simulink model "full_maneuver_platoon_new_strategy"  (R2019a)
settings: Solver=VariableStepAuto  StartTime=0.0  StopTime=70  FixedStep=0.1  MaxStep=0.05  RelTol=1e-3
libraries: simulink x97, dspsigops x7, powerlib_meascontrol x7, autolibshared x7
(part 6 of 7)

== system full_maneuver_platoon_new_strategy/p1/Vehicle Following During LC/Velocity Control ==
  velocity : Inport
  realInput : Inport  Port=2
  intReset : Inport  Port=3
  Anti-windup gain : Gain  Gain=velKp/velKi
  Integrator2 : Integrator  ExternalReset=falling
  Sum : Sum  Inputs=|+-
  Sum1 : Sum  Inputs=|-+
  Sum2 : Sum  Inputs=-+|
  Sum3 : Sum  Inputs=|++
  freeFlowVel : Constant  Value=freeFlowVel
  velKi : Gain  Gain=velKi
  velKp : Gain  Gain=velKp
  u : Outport
  wires:
  Sum/1 -> velKi/1, velKp/1
  velKp/1 -> Sum3/2
  velKi/1 -> Sum2/2
  Integrator2/1 -> Sum3/1
  velocity/1 -> Sum/2
  freeFlowVel/1 -> Sum/1
  intReset/1 -> Integrator2/2
  Sum3/1 -> Sum1/2, u/1
  Anti-windup gain/1 -> Sum2/1
  realInput/1 -> Sum1/1
  Sum1/1 -> Anti-windup gain/1
  Sum2/1 -> Integrator2/1

== system full_maneuver_platoon_new_strategy/p1/Virtual Vehicle Following/Compute Errors ==
  xf : Inport
  vf : Inport  Port=2
  xl : Inport  Port=3
  vl : Inport  Port=4
  lcFlag : Inport  Port=5
  Compare To Constant : simulink/Logic and Bit Operations/Compare To Constant  relop=<=  const=0  OutDataTypeStr=boolean
  Demux : Demux  Outputs=2
  Demux1 : Demux  Outputs=2
  Gain3 : Gain  Gain=velFilterGain/10
  Integrator : Integrator  InitialCondition=[h d0]
  Integrator1 : Integrator  InitialCondition=vx0
  Multiply : Product
  Mux : Mux  Inputs=2
  Mux1 : Mux  Inputs=2
  Product : Product
  Saturation : Saturate  UpperLimit=maxAcceleration  LowerLimit=minAcceleration
  Sum : Sum  Inputs=-+|
  Sum1 : Sum  Inputs=++|
  Sum2 : Sum  Inputs=+-|
  Sum3 : Sum  Inputs=|++
  Sum4 : Sum  Inputs=-+|
  Sum5 : Sum  Inputs=|+-
  Sum6 : Sum  Inputs=+-|
  Sum7 : Sum  Inputs=|++
  Sum8 : Sum  Inputs=|+-
  Switch : Switch  Criteria=u2 > Threshold
  d0 : Constant  Value=d0
  d0Lc : Constant  Value=d0Lc
  h : Constant  Value=h
  hFilterGain : Gain  Gain=hFilterGain
  hLc : Constant  Value=hLc
  vLen : Constant  Value=lr+lf
  eh : Outport
  ev : Outport  Port=2
  "gap " : Outport  Port=3
  unsafeFlag : Outport  Port=4
  wires:
  vl/1 -> Sum8/1
  Saturation/1 -> Integrator1/1
  Sum8/1 -> Gain3/1
  Gain3/1 -> Saturation/1
  Integrator1/1 -> Sum8/2, Sum4/2
  Sum4/1 -> ev/1
  d0Lc/1 -> Mux1/2
  hFilterGain/1 -> Integrator/1
  Demux/1 -> Multiply/2
  xf/1 -> Sum1/2
  Sum/1 -> Sum2/1, "gap "/1, Sum6/1  "gap"
  Multiply/1 -> Sum3/1
  Demux1/2 -> Sum7/2
  hLc/1 -> Mux1/1
  vLen/1 -> Sum1/1
  Demux/2 -> Sum3/2
  Switch/1 -> Sum5/1
  Sum5/1 -> hFilterGain/1
  vf/1 -> Multiply/1, Product/1, Sum4/1
  Sum1/1 -> Sum/1  "x (front bumber)"
  Sum3/1 -> Sum2/2  "desired  gap"
  h/1 -> Mux/1
  Product/1 -> Sum7/1
  xl/1 -> Sum/2
  lcFlag/1 -> Switch/2
  Sum2/1 -> eh/1
  Compare To Constant/1 -> unsafeFlag/1
  Demux1/1 -> Product/2
  Integrator/1 -> Sum5/2, Demux/1
  d0/1 -> Mux/2
  Mux1/1 -> Switch/1
  Sum7/1 -> Sum6/2  "safe  gap"
  Mux/1 -> Switch/3, Demux1/1  "min safe gap"
  Sum6/1 -> Compare To Constant/1

== system full_maneuver_platoon_new_strategy/p1/Virtual Vehicle Following/Velocity Control ==
  note: Velocity control
  intReset : Inport
  ev : Inport  Port=2
  Integrator2 : Integrator  ExternalReset=rising
  Sum3 : Sum
  velKi : Gain  Gain=velKi
  velKp : Gain  Gain=velKp
  Out1 : Outport
  wires:
  intReset/1 -> Integrator2/2
  ev/1 -> Integrator2/1, velKp/1
  velKp/1 -> Sum3/1
  Sum3/1 -> Out1/1
  velKi/1 -> Sum3/2
  Integrator2/1 -> velKi/1

== system full_maneuver_platoon_new_strategy/p1/Virtual Vehicle Following/Virtual Leader Following ==
  eh : Inport
  ev : Inport  Port=2
  realInput : Inport  Port=3
  Anti-windup gain : Gain  Gain=sqrt(Ki/Kd)
  Integrator : Integrator
  Kd : Gain  Gain=Kd
  Ki : Gain  Gain=Ki
  Kp : Gain  Gain=Kp
  Saturation1 : Saturate  UpperLimit=maxHeadwayError  LowerLimit=minHeadwayError
  Scope : Scope  NumInputPorts=4
  Sum : Sum  Inputs=|-+
  Sum1 : Sum  Inputs=+++
  Sum5 : Sum  Inputs=-+|
  u : Outport
  wires:
  Sum/1 -> Anti-windup gain/1
  realInput/1 -> Sum/1
  Sum1/1 -> u/1, Sum/2, Scope/4
  eh/1 -> Saturation1/1
  Saturation1/1 -> Ki/1, Kp/1
  Kd/1 -> Sum1/3, Scope/3
  Kp/1 -> Sum1/2, Scope/2
  Integrator/1 -> Sum1/1, Scope/1
  Sum5/1 -> Integrator/1
  Anti-windup gain/1 -> Sum5/1
  Ki/1 -> Sum5/2
  ev/1 -> Kd/1

== system full_maneuver_platoon_new_strategy/p1/followerErrors/gapToFollower ==
  xf : Inport
  vf : Inport  Port=2
  xl : Inport  Port=3
  Multiply : Product
  Sum : Sum  Inputs=-+|
  Sum1 : Sum  Inputs=++|
  Sum2 : Sum  Inputs=+-|
  Sum3 : Sum  Inputs=|++
  d0 : Constant  Value=d0
  h : Constant  Value=h
  vLen : Constant  Value=lr+lf
  eh : Outport
  "gap " : Outport  Port=2
  wires:
  d0/1 -> Sum3/2  "gap at  standstill"
  h/1 -> Multiply/2  "time headway"
  Sum2/1 -> eh/1
  xl/1 -> Sum/2
  Sum1/1 -> Sum/1  "x (front bumber)"
  vf/1 -> Multiply/1
  Sum3/1 -> Sum2/2  "desired  gap"
  xf/1 -> Sum1/2
  Sum/1 -> Sum2/1, "gap "/1  "gap"
  Multiply/1 -> Sum3/1
  vLen/1 -> Sum1/1

== system full_maneuver_platoon_new_strategy/p2/Lateral Control/Full State Observer ==
  note: yhat
  note: xhat
  measuredOutputs : Inport
  delta : Inport  Port=2
  Add1 : Sum  Inputs=|-+
  Gain : Gain  Gain=B  Multiplication=Matrix(K*u)
  Gain1 : Gain  Gain=C  Multiplication=Matrix(K*u)
  Gain2 : Gain  Gain=L  Multiplication=Matrix(K*u)
  Gain3 : Gain  Gain=A  Multiplication=Matrix(K*u)
  Integrator : Integrator  InitialCondition=[y0; 0; 0; 0]
  Signal Specification : SignalSpecification  Dimensions=[size(C,1) 1]
  Sum : Sum  Inputs=+++
  xhat : Outport
  wires:
  Gain2/1 -> Sum/1
  Signal Specification/1 -> Gain2/1
  Gain3/1 -> Sum/2
  Gain/1 -> Sum/3
  delta/1 -> Gain/1
  measuredOutputs/1 -> Add1/2
  Sum/1 -> Integrator/1
  Gain1/1 -> Add1/1
  Integrator/1 -> Gain1/1, Gain3/1, xhat/1
  Add1/1 -> Signal Specification/1

== system full_maneuver_platoon_new_strategy/p2/Lateral Control/Triggered Subsystem1 ==
  In1 : Inport
  Trigger : TriggerPort  VariantControl=Variant
  Out1 : Outport  InitialOutput=y0
  wires:
  In1/1 -> Out1/1

== system full_maneuver_platoon_new_strategy/p2/Regular Vehicle Following/Compute Errors ==
  xf : Inport
  vf : Inport  Port=2
  xl : Inport  Port=3
  vl : Inport  Port=4
  extraSpaceFlag : Inport  Port=5
  Compare To Constant : simulink/Logic and Bit Operations/Compare To Constant  relop=<  const=-0.1  OutDataTypeStr=boolean
  Demux : Demux  Outputs=2
  Demux1 : Demux  Outputs=2
  Gain3 : Gain  Gain=velFilterGain
  Integrator : Integrator  InitialCondition=[h d0]
  Integrator1 : Integrator  InitialCondition=vx0
  Multiply : Product
  Mux : Mux  Inputs=2
  Mux1 : Mux  Inputs=2
  Product : Product
  Saturation : Saturate  UpperLimit=maxAcceleration  LowerLimit=minAcceleration
  Sum : Sum  Inputs=-+|
  Sum1 : Sum  Inputs=++|
  Sum2 : Sum  Inputs=+-|
  Sum3 : Sum  Inputs=|++
  Sum4 : Sum  Inputs=-+|
  Sum5 : Sum  Inputs=|+-
  Sum6 : Sum  Inputs=+-|
  Sum7 : Sum  Inputs=|++
  Sum8 : Sum  Inputs=|+-
  Switch : Switch  Criteria=u2 > Threshold
  d0 : Constant  Value=d0
  d0Lc : Constant  Value=d0Lc
  h : Constant  Value=h
  hFilterGain : Gain  Gain=hFilterGain
  hLc : Constant  Value=hLc
  vLen : Constant  Value=lr+lf
  eh : Outport
  ev : Outport  Port=2
  "gap " : Outport  Port=3
  unsafeFlag : Outport  Port=4
  wires:
  Sum6/1 -> Compare To Constant/1
  Mux/1 -> Switch/3, Demux1/1  "min safe gap"
  Sum7/1 -> Sum6/2  "safe  gap"
  Mux1/1 -> Switch/1
  d0/1 -> Mux/2
  Integrator/1 -> Demux/1, Sum5/2
  Demux1/1 -> Product/2
  Compare To Constant/1 -> unsafeFlag/1
  Sum2/1 -> eh/1
  extraSpaceFlag/1 -> Switch/2
  xl/1 -> Sum/2
  Product/1 -> Sum7/1
  h/1 -> Mux/1
  Sum3/1 -> Sum2/2  "desired  gap"
  Sum1/1 -> Sum/1  "x (front bumber)"
  vf/1 -> Sum4/1, Product/1, Multiply/1
  Sum5/1 -> hFilterGain/1
  Switch/1 -> Sum5/1
  Demux/2 -> Sum3/2
  vLen/1 -> Sum1/1
  hLc/1 -> Mux1/1
  Demux1/2 -> Sum7/2
  Multiply/1 -> Sum3/1
  Sum/1 -> Sum6/1, "gap "/1, Sum2/1  "gap"
  xf/1 -> Sum1/2
  Demux/1 -> Multiply/2
  hFilterGain/1 -> Integrator/1
  d0Lc/1 -> Mux1/2
  vl/1 -> Sum8/1
  Sum4/1 -> ev/1
  Gain3/1 -> Saturation/1
  Saturation/1 -> Integrator1/1
  Integrator1/1 -> Sum4/2, Sum8/2
  Sum8/1 -> Gain3/1

== system full_maneuver_platoon_new_strategy/p2/Regular Vehicle Following/Free Flow Velocity Control ==
  ev : Inport
  realInput : Inport  Port=2
  intReset : Inport  Port=3
  Anti-windup gain : Gain  Gain=velKp/velKi
  Integrator2 : Integrator  ExternalReset=falling
  Sum1 : Sum  Inputs=|-+
  Sum2 : Sum  Inputs=-+|
  Sum3 : Sum  Inputs=|++
  velKi : Gain  Gain=velKi
  velKp : Gain  Gain=velKp
  u : Outport
  wires:
  ev/1 -> velKp/1, velKi/1
  velKp/1 -> Sum3/2
  velKi/1 -> Sum2/2
  Integrator2/1 -> Sum3/1
  intReset/1 -> Integrator2/2
  Sum3/1 -> Sum1/2, u/1
  Anti-windup gain/1 -> Sum2/1
  realInput/1 -> Sum1/1
  Sum1/1 -> Anti-windup gain/1
  Sum2/1 -> Integrator2/1

== system full_maneuver_platoon_new_strategy/p2/Regular Vehicle Following/Minimum Velocity Control ==
  ev : Inport
  realInput : Inport  Port=2
  intReset : Inport  Port=3
  Anti-windup gain : Gain  Gain=velKp/velKi
  Integrator2 : Integrator  ExternalReset=rising
  Sum1 : Sum  Inputs=|-+
  Sum2 : Sum  Inputs=-+|
  Sum3 : Sum  Inputs=|++
  velKi : Gain  Gain=velKi
  velKp : Gain  Gain=velKp
  u : Outport
  wires:
  ev/1 -> velKp/1, velKi/1
  velKp/1 -> Sum3/2
  velKi/1 -> Sum2/2
  Integrator2/1 -> Sum3/1
  intReset/1 -> Integrator2/2
  Sum3/1 -> Sum1/2, u/1
  Anti-windup gain/1 -> Sum2/1
  realInput/1 -> Sum1/1
  Sum1/1 -> Anti-windup gain/1
  Sum2/1 -> Integrator2/1

== system full_maneuver_platoon_new_strategy/p2/Regular Vehicle Following/Veh Following ==
  eh : Inport
  ev : Inport  Port=2
  realInput : Inport  Port=3
  intReset : Inport  Port=4
  Anti-windup gain : Gain  Gain=sqrt(Ki/Kd)
  Integrator : Integrator  ExternalReset=rising
  Kd : Gain  Gain=Kd
  Ki : Gain  Gain=Ki
  Kp : Gain  Gain=Kp
  Saturation1 : Saturate  UpperLimit=maxHeadwayError  LowerLimit=minHeadwayError
  Scope : Scope  NumInputPorts=4
  Sum : Sum  Inputs=|-+
  Sum1 : Sum  Inputs=+++
  Sum5 : Sum  Inputs=-+|
  u : Outport
  wires:
  ev/1 -> Kd/1
  Ki/1 -> Sum5/2
  Anti-windup gain/1 -> Sum5/1
  Sum5/1 -> Integrator/1
  Integrator/1 -> Sum1/1, Scope/1
  Kp/1 -> Sum1/2, Scope/2
  Kd/1 -> Scope/3, Sum1/3
  Saturation1/1 -> Kp/1, Ki/1
  eh/1 -> Saturation1/1
  Sum1/1 -> Sum/2, u/1, Scope/4
  realInput/1 -> Sum/1
  Sum/1 -> Anti-windup gain/1
  intReset/1 -> Integrator/2

== system full_maneuver_platoon_new_strategy/p2/Vehicle Following During LC/Compute Errors ==
  xf : Inport
  vf : Inport  Port=2
  xl : Inport  Port=3
  vl : Inport  Port=4
  extraSpaceFlag : Inport  Port=5
  Compare To Constant : simulink/Logic and Bit Operations/Compare To Constant  relop=<=  const=0  OutDataTypeStr=boolean
  Demux : Demux  Outputs=2
  Demux1 : Demux  Outputs=2
  Gain3 : Gain  Gain=velFilterGain
  Integrator : Integrator  InitialCondition=[h d0]
  Integrator1 : Integrator  InitialCondition=vx0
  Multiply : Product
  Mux : Mux  Inputs=2
  Mux1 : Mux  Inputs=2
  Product : Product
  Saturation : Saturate  UpperLimit=maxAcceleration  LowerLimit=minAcceleration
  Sum : Sum  Inputs=-+|
  Sum1 : Sum  Inputs=++|
  Sum2 : Sum  Inputs=+-|
  Sum3 : Sum  Inputs=|++
  Sum4 : Sum  Inputs=-+|
  Sum5 : Sum  Inputs=|+-
  Sum6 : Sum  Inputs=+-|
  Sum7 : Sum  Inputs=|++
  Sum8 : Sum  Inputs=|+-
  Switch : Switch  Criteria=u2 > Threshold
  d0 : Constant  Value=d0
  d0Lc : Constant  Value=d0Lc
  h : Constant  Value=h
  hFilterGain : Gain  Gain=hFilterGain
  hLc : Constant  Value=hLc
  vLen : Constant  Value=lr+lf
  eh : Outport
  ev : Outport  Port=2
  "gap " : Outport  Port=3
  unsafeFlag : Outport  Port=4
  wires:
  Sum4/1 -> ev/1
  d0Lc/1 -> Mux1/2
  hFilterGain/1 -> Integrator/1
  Demux/1 -> Multiply/2
  xf/1 -> Sum1/2
  Sum/1 -> Sum2/1, "gap "/1, Sum6/1  "gap"
  Multiply/1 -> Sum3/1
  Demux1/2 -> Sum7/2
  hLc/1 -> Mux1/1
  vLen/1 -> Sum1/1
  Demux/2 -> Sum3/2
  Switch/1 -> Sum5/1
  Sum5/1 -> hFilterGain/1
  vf/1 -> Multiply/1, Product/1, Sum4/1
  Sum1/1 -> Sum/1  "x (front bumber)"
  Sum3/1 -> Sum2/2  "desired  gap"
  h/1 -> Mux/1
  Product/1 -> Sum7/1
  xl/1 -> Sum/2
  extraSpaceFlag/1 -> Switch/2
  Sum2/1 -> eh/1
  Compare To Constant/1 -> unsafeFlag/1
  Demux1/1 -> Product/2
  Integrator/1 -> Sum5/2, Demux/1
  d0/1 -> Mux/2
  Mux1/1 -> Switch/1
  Sum7/1 -> Sum6/2  "safe  gap"
  Mux/1 -> Switch/3, Demux1/1  "min safe gap"
  Sum6/1 -> Compare To Constant/1
  Saturation/1 -> Integrator1/1
  Gain3/1 -> Saturation/1
  Integrator1/1 -> Sum4/2, Sum8/2
  Sum8/1 -> Gain3/1
  vl/1 -> Sum8/1

== system full_maneuver_platoon_new_strategy/p2/Vehicle Following During LC/Veh Following ==
  eh : Inport
  ev : Inport  Port=2
  realInput : Inport  Port=3
  intReset : Inport  Port=4
  Anti-windup gain : Gain  Gain=sqrt(Ki/Kd)
  Integrator : Integrator  ExternalReset=rising
  Kd : Gain  Gain=Kd
  Ki : Gain  Gain=Ki
  Kp : Gain  Gain=Kp
  Saturation1 : Saturate  UpperLimit=maxHeadwayError  LowerLimit=minHeadwayError
  Scope : Scope  NumInputPorts=4
  Sum : Sum  Inputs=|-+
  Sum1 : Sum  Inputs=+++
  Sum5 : Sum  Inputs=-+|
  u : Outport
  wires:
  intReset/1 -> Integrator/2
  Sum/1 -> Anti-windup gain/1
  realInput/1 -> Sum/1
  Sum1/1 -> Scope/4, u/1, Sum/2
  eh/1 -> Saturation1/1
  Saturation1/1 -> Ki/1, Kp/1
  Kd/1 -> Sum1/3, Scope/3
  Kp/1 -> Scope/2, Sum1/2
  Integrator/1 -> Scope/1, Sum1/1
  Sum5/1 -> Integrator/1
  Anti-windup gain/1 -> Sum5/1
  Ki/1 -> Sum5/2
  ev/1 -> Kd/1

== system full_maneuver_platoon_new_strategy/p2/Vehicle Following During LC/Velocity Control ==
  velocity : Inport
  realInput : Inport  Port=2
  intReset : Inport  Port=3
  Anti-windup gain : Gain  Gain=velKp/velKi
  Integrator2 : Integrator  ExternalReset=falling
  Sum : Sum  Inputs=|+-
  Sum1 : Sum  Inputs=|-+
  Sum2 : Sum  Inputs=-+|
  Sum3 : Sum  Inputs=|++
  freeFlowVel : Constant  Value=freeFlowVel
  velKi : Gain  Gain=velKi
  velKp : Gain  Gain=velKp
  u : Outport
  wires:
  Sum2/1 -> Integrator2/1
  Sum1/1 -> Anti-windup gain/1
  realInput/1 -> Sum1/1
  Anti-windup gain/1 -> Sum2/1
  Sum3/1 -> u/1, Sum1/2
  intReset/1 -> Integrator2/2
  freeFlowVel/1 -> Sum/1
  velocity/1 -> Sum/2
  Integrator2/1 -> Sum3/1
  velKi/1 -> Sum2/2
  velKp/1 -> Sum3/2
  Sum/1 -> velKp/1, velKi/1

== system full_maneuver_platoon_new_strategy/p2/Virtual Vehicle Following/Compute Errors ==
  xf : Inport
  vf : Inport  Port=2
  xl : Inport  Port=3
  vl : Inport  Port=4
  lcFlag : Inport  Port=5
  Compare To Constant : simulink/Logic and Bit Operations/Compare To Constant  relop=<=  const=0  OutDataTypeStr=boolean
  Demux : Demux  Outputs=2
  Demux1 : Demux  Outputs=2
  Gain3 : Gain  Gain=velFilterGain/10
  Integrator : Integrator  InitialCondition=[h d0]
  Integrator1 : Integrator  InitialCondition=vx0
  Multiply : Product
  Mux : Mux  Inputs=2
  Mux1 : Mux  Inputs=2
  Product : Product
  Saturation : Saturate  UpperLimit=maxAcceleration  LowerLimit=minAcceleration
  Sum : Sum  Inputs=-+|
  Sum1 : Sum  Inputs=++|
  Sum2 : Sum  Inputs=+-|
  Sum3 : Sum  Inputs=|++
  Sum4 : Sum  Inputs=-+|
  Sum5 : Sum  Inputs=|+-
  Sum6 : Sum  Inputs=+-|
  Sum7 : Sum  Inputs=|++
  Sum8 : Sum  Inputs=|+-
  Switch : Switch  Criteria=u2 > Threshold
  d0 : Constant  Value=d0
  d0Lc : Constant  Value=d0Lc
  h : Constant  Value=h
  hFilterGain : Gain  Gain=hFilterGain
  hLc : Constant  Value=hLc
  vLen : Constant  Value=lr+lf
  eh : Outport
  ev : Outport  Port=2
  "gap " : Outport  Port=3
  unsafeFlag : Outport  Port=4
  wires:
  Sum6/1 -> Compare To Constant/1
  Mux/1 -> Demux1/1, Switch/3  "min safe gap"
  Sum7/1 -> Sum6/2  "safe  gap"
  Mux1/1 -> Switch/1
  d0/1 -> Mux/2
  Integrator/1 -> Demux/1, Sum5/2
  Demux1/1 -> Product/2
  Compare To Constant/1 -> unsafeFlag/1
  Sum2/1 -> eh/1
  lcFlag/1 -> Switch/2
  xl/1 -> Sum/2
  Product/1 -> Sum7/1
  h/1 -> Mux/1
  Sum3/1 -> Sum2/2  "desired  gap"
  Sum1/1 -> Sum/1  "x (front bumber)"
  vf/1 -> Sum4/1, Product/1, Multiply/1
  Sum5/1 -> hFilterGain/1
  Switch/1 -> Sum5/1
  Demux/2 -> Sum3/2
  vLen/1 -> Sum1/1
  hLc/1 -> Mux1/1
  Demux1/2 -> Sum7/2
  Multiply/1 -> Sum3/1
  Sum/1 -> Sum6/1, "gap "/1, Sum2/1  "gap"
  xf/1 -> Sum1/2
  Demux/1 -> Multiply/2
  hFilterGain/1 -> Integrator/1
  d0Lc/1 -> Mux1/2
  Sum4/1 -> ev/1
  Integrator1/1 -> Sum4/2, Sum8/2
  Gain3/1 -> Saturation/1
  Sum8/1 -> Gain3/1
  Saturation/1 -> Integrator1/1
  vl/1 -> Sum8/1

== system full_maneuver_platoon_new_strategy/p2/Virtual Vehicle Following/Velocity Control ==
  note: Velocity control
  intReset : Inport
  ev : Inport  Port=2
  Integrator2 : Integrator  ExternalReset=rising
  Sum3 : Sum
  velKi : Gain  Gain=velKi
  velKp : Gain  Gain=velKp
  Out1 : Outport
  wires:
  Integrator2/1 -> velKi/1
  velKi/1 -> Sum3/2
  Sum3/1 -> Out1/1
  velKp/1 -> Sum3/1
  ev/1 -> velKp/1, Integrator2/1
  intReset/1 -> Integrator2/2

== system full_maneuver_platoon_new_strategy/p2/Virtual Vehicle Following/Virtual Leader Following ==
  eh : Inport
  ev : Inport  Port=2
  realInput : Inport  Port=3
  Anti-windup gain : Gain  Gain=sqrt(Ki/Kd)
  Integrator : Integrator
  Kd : Gain  Gain=Kd
  Ki : Gain  Gain=Ki
  Kp : Gain  Gain=Kp
  Saturation1 : Saturate  UpperLimit=maxHeadwayError  LowerLimit=minHeadwayError
  Scope : Scope  NumInputPorts=4
  Sum : Sum  Inputs=|-+
  Sum1 : Sum  Inputs=+++
  Sum5 : Sum  Inputs=-+|
  u : Outport
  wires:
  ev/1 -> Kd/1
  Ki/1 -> Sum5/2
  Anti-windup gain/1 -> Sum5/1
  Sum5/1 -> Integrator/1
  Integrator/1 -> Scope/1, Sum1/1
  Kp/1 -> Scope/2, Sum1/2
  Kd/1 -> Scope/3, Sum1/3
  Saturation1/1 -> Kp/1, Ki/1
  eh/1 -> Saturation1/1
  Sum1/1 -> Scope/4, Sum/2, u/1
  realInput/1 -> Sum/1
  Sum/1 -> Anti-windup gain/1

== system full_maneuver_platoon_new_strategy/p2/followerErrors/gapToFollower ==
  xf : Inport
  vf : Inport  Port=2
  xl : Inport  Port=3
  Multiply : Product
  Sum : Sum  Inputs=-+|
  Sum1 : Sum  Inputs=++|
  Sum2 : Sum  Inputs=+-|
  Sum3 : Sum  Inputs=|++
  d0 : Constant  Value=d0
  h : Constant  Value=h
  vLen : Constant  Value=lr+lf
  eh : Outport
  "gap " : Outport  Port=2
  wires:
  vLen/1 -> Sum1/1
  Multiply/1 -> Sum3/1
  Sum/1 -> "gap "/1, Sum2/1  "gap"
  xf/1 -> Sum1/2
  Sum3/1 -> Sum2/2  "desired  gap"
  vf/1 -> Multiply/1
  Sum1/1 -> Sum/1  "x (front bumber)"
  xl/1 -> Sum/2
  Sum2/1 -> eh/1
  h/1 -> Multiply/2  "time headway"
  d0/1 -> Sum3/2  "gap at  standstill"

== system full_maneuver_platoon_new_strategy/p3/Lateral Control/Full State Observer ==
  note: xhat
  note: yhat
  measuredOutputs : Inport
  delta : Inport  Port=2
  Add1 : Sum  Inputs=|-+
  Gain : Gain  Gain=B  Multiplication=Matrix(K*u)
  Gain1 : Gain  Gain=C  Multiplication=Matrix(K*u)
  Gain2 : Gain  Gain=L  Multiplication=Matrix(K*u)
  Gain3 : Gain  Gain=A  Multiplication=Matrix(K*u)
  Integrator : Integrator  InitialCondition=[y0; 0; 0; 0]
  Signal Specification : SignalSpecification  Dimensions=[size(C,1) 1]
  Sum : Sum  Inputs=+++
  xhat : Outport
  wires:
  Add1/1 -> Signal Specification/1
  Integrator/1 -> xhat/1, Gain3/1, Gain1/1
  Gain1/1 -> Add1/1
  Sum/1 -> Integrator/1
  measuredOutputs/1 -> Add1/2
  delta/1 -> Gain/1
  Gain/1 -> Sum/3
  Gain3/1 -> Sum/2
  Signal Specification/1 -> Gain2/1
  Gain2/1 -> Sum/1

== system full_maneuver_platoon_new_strategy/p3/Lateral Control/Triggered Subsystem1 ==
  In1 : Inport
  Trigger : TriggerPort  VariantControl=Variant
  Out1 : Outport  InitialOutput=y0
  wires:
  In1/1 -> Out1/1

== system full_maneuver_platoon_new_strategy/p3/Regular Vehicle Following/Compute Errors ==
  xf : Inport
  vf : Inport  Port=2
  xl : Inport  Port=3
  vl : Inport  Port=4
  extraSpaceFlag : Inport  Port=5
  Compare To Constant : simulink/Logic and Bit Operations/Compare To Constant  relop=<  const=-0.1  OutDataTypeStr=boolean
  Demux : Demux  Outputs=2
  Demux1 : Demux  Outputs=2
  Gain3 : Gain  Gain=velFilterGain
  Integrator : Integrator  InitialCondition=[h d0]
  Integrator1 : Integrator  InitialCondition=vx0
  Multiply : Product
  Mux : Mux  Inputs=2
  Mux1 : Mux  Inputs=2
  Product : Product
  Saturation : Saturate  UpperLimit=maxAcceleration  LowerLimit=minAcceleration
  Sum : Sum  Inputs=-+|
  Sum1 : Sum  Inputs=++|
  Sum2 : Sum  Inputs=+-|
  Sum3 : Sum  Inputs=|++
  Sum4 : Sum  Inputs=-+|
  Sum5 : Sum  Inputs=|+-
  Sum6 : Sum  Inputs=+-|
  Sum7 : Sum  Inputs=|++
  Sum8 : Sum  Inputs=|+-
  Switch : Switch  Criteria=u2 > Threshold
  d0 : Constant  Value=d0
  d0Lc : Constant  Value=d0Lc
  h : Constant  Value=h
  hFilterGain : Gain  Gain=hFilterGain
  hLc : Constant  Value=hLc
  vLen : Constant  Value=lr+lf
  eh : Outport
  ev : Outport  Port=2
  "gap " : Outport  Port=3
  unsafeFlag : Outport  Port=4
  wires:
  Sum8/1 -> Gain3/1
  Integrator1/1 -> Sum8/2, Sum4/2
  Saturation/1 -> Integrator1/1
  Gain3/1 -> Saturation/1
  Sum4/1 -> ev/1
  vl/1 -> Sum8/1
  d0Lc/1 -> Mux1/2
  hFilterGain/1 -> Integrator/1
  Demux/1 -> Multiply/2
  xf/1 -> Sum1/2
  Sum/1 -> Sum2/1, "gap "/1, Sum6/1  "gap"
  Multiply/1 -> Sum3/1
  Demux1/2 -> Sum7/2
  hLc/1 -> Mux1/1
  vLen/1 -> Sum1/1
  Demux/2 -> Sum3/2
  Switch/1 -> Sum5/1
  Sum5/1 -> hFilterGain/1
  vf/1 -> Multiply/1, Product/1, Sum4/1
  Sum1/1 -> Sum/1  "x (front bumber)"
  Sum3/1 -> Sum2/2  "desired  gap"
  h/1 -> Mux/1
  Product/1 -> Sum7/1
  xl/1 -> Sum/2
  extraSpaceFlag/1 -> Switch/2
  Sum2/1 -> eh/1
  Compare To Constant/1 -> unsafeFlag/1
  Demux1/1 -> Product/2
  Integrator/1 -> Sum5/2, Demux/1
  d0/1 -> Mux/2
  Mux1/1 -> Switch/1
  Sum7/1 -> Sum6/2  "safe  gap"
  Mux/1 -> Demux1/1, Switch/3  "min safe gap"
  Sum6/1 -> Compare To Constant/1

== system full_maneuver_platoon_new_strategy/p3/Regular Vehicle Following/Free Flow Velocity Control ==
  ev : Inport
  realInput : Inport  Port=2
  intReset : Inport  Port=3
  Anti-windup gain : Gain  Gain=velKp/velKi
  Integrator2 : Integrator  ExternalReset=falling
  Sum1 : Sum  Inputs=|-+
  Sum2 : Sum  Inputs=-+|
  Sum3 : Sum  Inputs=|++
  velKi : Gain  Gain=velKi
  velKp : Gain  Gain=velKp
  u : Outport
  wires:
  Sum2/1 -> Integrator2/1
  Sum1/1 -> Anti-windup gain/1
  realInput/1 -> Sum1/1
  Anti-windup gain/1 -> Sum2/1
  Sum3/1 -> u/1, Sum1/2
  intReset/1 -> Integrator2/2
  Integrator2/1 -> Sum3/1
  velKi/1 -> Sum2/2
  velKp/1 -> Sum3/2
  ev/1 -> velKi/1, velKp/1

== system full_maneuver_platoon_new_strategy/p3/Regular Vehicle Following/Minimum Velocity Control ==
  ev : Inport
  realInput : Inport  Port=2
  intReset : Inport  Port=3
  Anti-windup gain : Gain  Gain=velKp/velKi
  Integrator2 : Integrator  ExternalReset=rising
  Sum1 : Sum  Inputs=|-+
  Sum2 : Sum  Inputs=-+|
  Sum3 : Sum  Inputs=|++
  velKi : Gain  Gain=velKi
  velKp : Gain  Gain=velKp
  u : Outport
  wires:
  Sum2/1 -> Integrator2/1
  Sum1/1 -> Anti-windup gain/1
  realInput/1 -> Sum1/1
  Anti-windup gain/1 -> Sum2/1
  Sum3/1 -> u/1, Sum1/2
  intReset/1 -> Integrator2/2
  Integrator2/1 -> Sum3/1
  velKi/1 -> Sum2/2
  velKp/1 -> Sum3/2
  ev/1 -> velKi/1, velKp/1

== system full_maneuver_platoon_new_strategy/p3/Regular Vehicle Following/Veh Following ==
  eh : Inport
  ev : Inport  Port=2
  realInput : Inport  Port=3
  intReset : Inport  Port=4
  Anti-windup gain : Gain  Gain=sqrt(Ki/Kd)
  Integrator : Integrator  ExternalReset=rising
  Kd : Gain  Gain=Kd
  Ki : Gain  Gain=Ki
  Kp : Gain  Gain=Kp
  Saturation1 : Saturate  UpperLimit=maxHeadwayError  LowerLimit=minHeadwayError
  Scope : Scope  NumInputPorts=4
  Sum : Sum  Inputs=|-+
  Sum1 : Sum  Inputs=+++
  Sum5 : Sum  Inputs=-+|
  u : Outport
  wires:
  intReset/1 -> Integrator/2
  Sum/1 -> Anti-windup gain/1
  realInput/1 -> Sum/1
  Sum1/1 -> Scope/4, u/1, Sum/2
  eh/1 -> Saturation1/1
  Saturation1/1 -> Ki/1, Kp/1
  Kd/1 -> Sum1/3, Scope/3
  Kp/1 -> Scope/2, Sum1/2
  Integrator/1 -> Scope/1, Sum1/1
  Sum5/1 -> Integrator/1
  Anti-windup gain/1 -> Sum5/1
  Ki/1 -> Sum5/2
  ev/1 -> Kd/1

== system full_maneuver_platoon_new_strategy/p3/Vehicle Following During LC/Compute Errors ==
  xf : Inport
  vf : Inport  Port=2
  xl : Inport  Port=3
  vl : Inport  Port=4
  extraSpaceFlag : Inport  Port=5
  Compare To Constant : simulink/Logic and Bit Operations/Compare To Constant  relop=<=  const=0  OutDataTypeStr=boolean
  Demux : Demux  Outputs=2
  Demux1 : Demux  Outputs=2
  Gain3 : Gain  Gain=velFilterGain
  Integrator : Integrator  InitialCondition=[h d0]
  Integrator1 : Integrator  InitialCondition=vx0
  Multiply : Product
  Mux : Mux  Inputs=2
  Mux1 : Mux  Inputs=2
  Product : Product
  Saturation : Saturate  UpperLimit=maxAcceleration  LowerLimit=minAcceleration
  Sum : Sum  Inputs=-+|
  Sum1 : Sum  Inputs=++|
  Sum2 : Sum  Inputs=+-|
  Sum3 : Sum  Inputs=|++
  Sum4 : Sum  Inputs=-+|
  Sum5 : Sum  Inputs=|+-
  Sum6 : Sum  Inputs=+-|
  Sum7 : Sum  Inputs=|++
  Sum8 : Sum  Inputs=|+-
  Switch : Switch  Criteria=u2 > Threshold
  d0 : Constant  Value=d0
  d0Lc : Constant  Value=d0Lc
  h : Constant  Value=h
  hFilterGain : Gain  Gain=hFilterGain
  hLc : Constant  Value=hLc
  vLen : Constant  Value=lr+lf
  eh : Outport
  ev : Outport  Port=2
  "gap " : Outport  Port=3
  unsafeFlag : Outport  Port=4
  wires:
  vl/1 -> Sum8/1
  Sum8/1 -> Gain3/1
  Integrator1/1 -> Sum8/2, Sum4/2
  Gain3/1 -> Saturation/1
  Saturation/1 -> Integrator1/1
  Sum6/1 -> Compare To Constant/1
  Mux/1 -> Demux1/1, Switch/3  "min safe gap"
  Sum7/1 -> Sum6/2  "safe  gap"
  Mux1/1 -> Switch/1
  d0/1 -> Mux/2
  Integrator/1 -> Demux/1, Sum5/2
  Demux1/1 -> Product/2
  Compare To Constant/1 -> unsafeFlag/1
  Sum2/1 -> eh/1
  extraSpaceFlag/1 -> Switch/2
  xl/1 -> Sum/2
  Product/1 -> Sum7/1
  h/1 -> Mux/1
  Sum3/1 -> Sum2/2  "desired  gap"
  Sum1/1 -> Sum/1  "x (front bumber)"
  vf/1 -> Sum4/1, Product/1, Multiply/1
  Sum5/1 -> hFilterGain/1
  Switch/1 -> Sum5/1
  Demux/2 -> Sum3/2
  vLen/1 -> Sum1/1
  hLc/1 -> Mux1/1
  Demux1/2 -> Sum7/2
  Multiply/1 -> Sum3/1
  Sum/1 -> Sum6/1, "gap "/1, Sum2/1  "gap"
  xf/1 -> Sum1/2
  Demux/1 -> Multiply/2
  hFilterGain/1 -> Integrator/1
  d0Lc/1 -> Mux1/2
  Sum4/1 -> ev/1

== system full_maneuver_platoon_new_strategy/p3/Vehicle Following During LC/Veh Following ==
  eh : Inport
  ev : Inport  Port=2
  realInput : Inport  Port=3
  intReset : Inport  Port=4
  Anti-windup gain : Gain  Gain=sqrt(Ki/Kd)
  Integrator : Integrator  ExternalReset=rising
  Kd : Gain  Gain=Kd
  Ki : Gain  Gain=Ki
  Kp : Gain  Gain=Kp
  Saturation1 : Saturate  UpperLimit=maxHeadwayError  LowerLimit=minHeadwayError
  Scope : Scope  NumInputPorts=4
  Sum : Sum  Inputs=|-+
  Sum1 : Sum  Inputs=+++
  Sum5 : Sum  Inputs=-+|
  u : Outport
  wires:
  ev/1 -> Kd/1
  Ki/1 -> Sum5/2
  Anti-windup gain/1 -> Sum5/1
  Sum5/1 -> Integrator/1
  Integrator/1 -> Sum1/1, Scope/1
  Kp/1 -> Sum1/2, Scope/2
  Kd/1 -> Scope/3, Sum1/3
  Saturation1/1 -> Kp/1, Ki/1
  eh/1 -> Saturation1/1
  Sum1/1 -> Sum/2, u/1, Scope/4
  realInput/1 -> Sum/1
  Sum/1 -> Anti-windup gain/1
  intReset/1 -> Integrator/2

== system full_maneuver_platoon_new_strategy/p3/Vehicle Following During LC/Velocity Control ==
  velocity : Inport
  realInput : Inport  Port=2
  intReset : Inport  Port=3
  Anti-windup gain : Gain  Gain=velKp/velKi
  Integrator2 : Integrator  ExternalReset=falling
  Sum : Sum  Inputs=|+-
  Sum1 : Sum  Inputs=|-+
  Sum2 : Sum  Inputs=-+|
  Sum3 : Sum  Inputs=|++
  freeFlowVel : Constant  Value=freeFlowVel
  velKi : Gain  Gain=velKi
  velKp : Gain  Gain=velKp
  u : Outport
  wires:
  Sum/1 -> velKi/1, velKp/1
  velKp/1 -> Sum3/2
  velKi/1 -> Sum2/2
  Integrator2/1 -> Sum3/1
  velocity/1 -> Sum/2
  freeFlowVel/1 -> Sum/1
  intReset/1 -> Integrator2/2
  Sum3/1 -> Sum1/2, u/1
  Anti-windup gain/1 -> Sum2/1
  realInput/1 -> Sum1/1
  Sum1/1 -> Anti-windup gain/1
  Sum2/1 -> Integrator2/1

== system full_maneuver_platoon_new_strategy/p3/Virtual Vehicle Following/Compute Errors ==
  xf : Inport
  vf : Inport  Port=2
  xl : Inport  Port=3
  vl : Inport  Port=4
  lcFlag : Inport  Port=5
  Compare To Constant : simulink/Logic and Bit Operations/Compare To Constant  relop=<=  const=0  OutDataTypeStr=boolean
  Demux : Demux  Outputs=2
  Demux1 : Demux  Outputs=2
  Gain3 : Gain  Gain=velFilterGain/10
  Integrator : Integrator  InitialCondition=[h d0]
  Integrator1 : Integrator  InitialCondition=vx0
  Multiply : Product
  Mux : Mux  Inputs=2
  Mux1 : Mux  Inputs=2
  Product : Product
  Saturation : Saturate  UpperLimit=maxAcceleration  LowerLimit=minAcceleration
  Sum : Sum  Inputs=-+|
  Sum1 : Sum  Inputs=++|
  Sum2 : Sum  Inputs=+-|
  Sum3 : Sum  Inputs=|++
  Sum4 : Sum  Inputs=-+|
  Sum5 : Sum  Inputs=|+-
  Sum6 : Sum  Inputs=+-|
  Sum7 : Sum  Inputs=|++
  Sum8 : Sum  Inputs=|+-
  Switch : Switch  Criteria=u2 > Threshold
  d0 : Constant  Value=d0
  d0Lc : Constant  Value=d0Lc
  h : Constant  Value=h
  hFilterGain : Gain  Gain=hFilterGain
  hLc : Constant  Value=hLc
  vLen : Constant  Value=lr+lf
  eh : Outport
  ev : Outport  Port=2
  "gap " : Outport  Port=3
  unsafeFlag : Outport  Port=4
  wires:
  vl/1 -> Sum8/1
  Saturation/1 -> Integrator1/1
  Sum8/1 -> Gain3/1
  Gain3/1 -> Saturation/1
  Integrator1/1 -> Sum8/2, Sum4/2
  Sum4/1 -> ev/1
  d0Lc/1 -> Mux1/2
  hFilterGain/1 -> Integrator/1
  Demux/1 -> Multiply/2
  xf/1 -> Sum1/2
  Sum/1 -> Sum2/1, "gap "/1, Sum6/1  "gap"
  Multiply/1 -> Sum3/1
  Demux1/2 -> Sum7/2
  hLc/1 -> Mux1/1
  vLen/1 -> Sum1/1
  Demux/2 -> Sum3/2
  Switch/1 -> Sum5/1
  Sum5/1 -> hFilterGain/1
  vf/1 -> Multiply/1, Product/1, Sum4/1
  Sum1/1 -> Sum/1  "x (front bumber)"
  Sum3/1 -> Sum2/2  "desired  gap"
  h/1 -> Mux/1
  Product/1 -> Sum7/1
  xl/1 -> Sum/2
  lcFlag/1 -> Switch/2
  Sum2/1 -> eh/1
  Compare To Constant/1 -> unsafeFlag/1
  Demux1/1 -> Product/2
  Integrator/1 -> Sum5/2, Demux/1
  d0/1 -> Mux/2
  Mux1/1 -> Switch/1
  Sum7/1 -> Sum6/2  "safe  gap"
  Mux/1 -> Switch/3, Demux1/1  "min safe gap"
  Sum6/1 -> Compare To Constant/1

== system full_maneuver_platoon_new_strategy/p3/Virtual Vehicle Following/Velocity Control ==
  note: Velocity control
  intReset : Inport
  ev : Inport  Port=2
  Integrator2 : Integrator  ExternalReset=rising
  Sum3 : Sum
  velKi : Gain  Gain=velKi
  velKp : Gain  Gain=velKp
  Out1 : Outport
  wires:
  intReset/1 -> Integrator2/2
  ev/1 -> Integrator2/1, velKp/1
  velKp/1 -> Sum3/1
  Sum3/1 -> Out1/1
  velKi/1 -> Sum3/2
  Integrator2/1 -> velKi/1

== system full_maneuver_platoon_new_strategy/p3/Virtual Vehicle Following/Virtual Leader Following ==
  eh : Inport
  ev : Inport  Port=2
  realInput : Inport  Port=3
  Anti-windup gain : Gain  Gain=sqrt(Ki/Kd)
  Integrator : Integrator
  Kd : Gain  Gain=Kd
  Ki : Gain  Gain=Ki
  Kp : Gain  Gain=Kp
  Saturation1 : Saturate  UpperLimit=maxHeadwayError  LowerLimit=minHeadwayError
  Scope : Scope  NumInputPorts=4
  Sum : Sum  Inputs=|-+
  Sum1 : Sum  Inputs=+++
  Sum5 : Sum  Inputs=-+|
  u : Outport
  wires:
  Sum/1 -> Anti-windup gain/1
  realInput/1 -> Sum/1
  Sum1/1 -> u/1, Sum/2, Scope/4
  eh/1 -> Saturation1/1
  Saturation1/1 -> Ki/1, Kp/1
  Kd/1 -> Sum1/3, Scope/3
  Kp/1 -> Sum1/2, Scope/2
  Integrator/1 -> Sum1/1, Scope/1
  Sum5/1 -> Integrator/1
  Anti-windup gain/1 -> Sum5/1
  Ki/1 -> Sum5/2
  ev/1 -> Kd/1

== system full_maneuver_platoon_new_strategy/p3/followerErrors/gapToFollower ==
  xf : Inport
  vf : Inport  Port=2
  xl : Inport  Port=3
  Multiply : Product
  Sum : Sum  Inputs=-+|
  Sum1 : Sum  Inputs=++|
  Sum2 : Sum  Inputs=+-|
  Sum3 : Sum  Inputs=|++
  d0 : Constant  Value=d0
  h : Constant  Value=h
  vLen : Constant  Value=lr+lf
  eh : Outport
  "gap " : Outport  Port=2
  wires:
  d0/1 -> Sum3/2  "gap at  standstill"
  h/1 -> Multiply/2  "time headway"
  Sum2/1 -> eh/1
  xl/1 -> Sum/2
  Sum1/1 -> Sum/1  "x (front bumber)"
  vf/1 -> Multiply/1
  Sum3/1 -> Sum2/2  "desired  gap"
  xf/1 -> Sum1/2
  Sum/1 -> Sum2/1, "gap "/1  "gap"
  Multiply/1 -> Sum3/1
  vLen/1 -> Sum1/1

== stateflow chart full_maneuver_platoon_new_strategy/Fd/ControlChoice ==
  state RegVehFoll
    entry:
    state = 1;
    during:
    data = regVehFollData;
  state AdjForLaneChange
    entry:
    state = 2;
    during:
    if leaderInRange
    data = min(regVehFollData, longAdjustmentData);
    else
    data = longAdjustmentData;
    end
  state LaneChanging
    entry:
    state = 3;
    during:
    if leaderInRange
    data = min(regVehFollData, laneChangingData);
    else
    data = laneChangingData;
    end
  (default) -> RegVehFoll
  LaneChanging -> RegVehFoll : [laneChangeDone]
  RegVehFoll -> LaneChanging [order 2] : [laneChangeStarted && ~laneChangeDone]
  RegVehFoll -> AdjForLaneChange [order 1] : [startAdjustment && ~laneChangeStarted]
  AdjForLaneChange -> LaneChanging : [laneChangeStarted]
  data: regVehFollData input; longAdjustmentData input; laneChangingData input; startAdjustment input size=1; data output; laneChangeStarted input; state output; laneChangeDone input; leaderInRange input

== stateflow chart full_maneuver_platoon_new_strategy/p1/ControlChoice ==
  state RegVehFoll
    entry:
    state = 1;
    during:
    data = regVehFollData;
  state AdjForLaneChange
    entry:
    state = 2;
    during:
    if leaderInRange
    data = min(regVehFollData, longAdjustmentData);
    else
    data = longAdjustmentData;
    end
  state LaneChanging
    entry:
    state = 3;
    during:
    if leaderInRange
    data = min(regVehFollData, laneChangingData);
    else
    data = laneChangingData;
    end
  (default) -> RegVehFoll
  LaneChanging -> RegVehFoll : [laneChangeDone]
  RegVehFoll -> LaneChanging [order 2] : [laneChangeStarted && ~laneChangeDone]
  RegVehFoll -> AdjForLaneChange [order 1] : [startAdjustment && ~laneChangeStarted]
  AdjForLaneChange -> LaneChanging : [laneChangeStarted]
  data: regVehFollData input; longAdjustmentData input; laneChangingData input; startAdjustment input size=1; data output; laneChangeStarted input; state output; laneChangeDone input; leaderInRange input

== matlab function full_maneuver_platoon_new_strategy/Fd/MATLAB Function ==
  data: leader output Bus: vehStatesBus; ego input Bus: vehStatesBus; allVehicles input; indices output; lcFlag input
function [leader, indices] = findLeader(ego, allVehicles, lcFlag)

nv = length(allVehicles);

leaderIdx = -1;

farAwayVehicle.X = ego.X + 10^4;
farAwayVehicle.Y = ego.Y;
farAwayVehicle.Xdot = ego.Xdot;
farAwayVehicle.u = 0;

leader = farAwayVehicle;

% For non lane changing vehicles, the leader is whoever is longitudinally
% closer and with any part of the body in the same lane
if ~lcFlag
    for n = 1:nv
        if allVehicles(n).X>ego.X && allVehicles(n).X<leader.X
            if abs(allVehicles(n).Y - ego.Y)<=2.7 % 1.8 (half lane) + 0.9 (half veh width)
                leader = allVehicles(n);
                leaderIdx=n;
            end
        end
    end
% For lane changing vehicles, we want to keep the original leader until the
% ego vehicle is out of the lane
else
    for n = 1:nv
        if allVehicles(n).X>ego.X && allVehicles(n).X<leader.X
            if abs(allVehicles(n).Y - ego.Y)<=1.9 % 1.8 (half lane) + 0.9 (half veh width)
                leader = allVehicles(n);
                leaderIdx=n;
            end
        end
    end
end

indices = leaderIdx;

== stateflow chart full_maneuver_platoon_new_strategy/Fd/Regular Vehicle Following/Chart ==
  state VehFollowing
    during:
    u = uVehFoll;
    state = 0;
  state SpeedControl
    during:
    u = uVelControl;
    state = 1;
  (default) -> VehFollowing
  SpeedControl -> VehFollowing : [leaderWithinRange==1]
  VehFollowing -> SpeedControl : [leaderWithinRange==0]
  data: state output size=1; u output size=1; leaderWithinRange input size=1; uVehFoll input size=1; uVelControl input double

== stateflow chart full_maneuver_platoon_new_strategy/Ld/ControlChoice ==
  state RegVehFoll
    entry:
    state = 1;
    during:
    data = regVehFollData;
  state AdjForLaneChange
    entry:
    state = 2;
    during:
    data = min(regVehFollData, longAdjustmentData);
  state LaneChanging
    entry:
    state = 3;
    during:
    data = min(regVehFollData, laneChangingData);
  (default) -> RegVehFoll
  LaneChanging -> RegVehFoll : [laneChangeDone]
  RegVehFoll -> LaneChanging [order 2] : [laneChangeStarted && ~laneChangeDone]
  RegVehFoll -> AdjForLaneChange [order 1] : [startAdjustment && ~laneChangeStarted]
  AdjForLaneChange -> LaneChanging : [laneChangeStarted==1]
  data: regVehFollData input; longAdjustmentData input; laneChangingData input; startAdjustment input size=1; data output; laneChangeStarted input; state output; laneChangeDone input

== matlab function full_maneuver_platoon_new_strategy/Ld/MATLAB Function ==
  data: leader output Bus: vehStatesBus; ego input Bus: vehStatesBus; allVehicles input; indices output
function [leader, indices] = findLeader(ego, allVehicles)

nv = length(allVehicles);

leaderIdx = -1;

farAwayVehicle.X = ego.X + 10^4;
farAwayVehicle.Y = ego.Y;
farAwayVehicle.Xdot = ego.Xdot;
farAwayVehicle.u = 0;

leader = farAwayVehicle;

for n = 1:nv
    if allVehicles(n).X>ego.X && allVehicles(n).X<leader.X
        if abs(allVehicles(n).Y - ego.Y)<=2.7 % 1.8 (half lane) + 0.9 (half veh width)
            leader = allVehicles(n);
            leaderIdx=n;
        end
    end
end

indices = leaderIdx;

== stateflow chart full_maneuver_platoon_new_strategy/Ld/Regular Vehicle Following/Chart ==
  state VehFollowing
    during:
    u = uVehFoll;
    state = 0;
  state SpeedControl
    during:
    u = uVelControl;
    state = 1;
  (default) -> VehFollowing
  SpeedControl -> VehFollowing : [leaderWithinRange==1]
  VehFollowing -> SpeedControl : [leaderWithinRange==0]
  data: state output size=1; u output size=1; leaderWithinRange input size=1; uVehFoll input size=1; uVelControl input double

== stateflow chart full_maneuver_platoon_new_strategy/Lo/ControlChoice ==
  state RegVehFoll
    entry:
    state = 1;
    during:
    data = regVehFollData;
  state AdjForLaneChange
    entry:
    state = 2;
    during:
    data = min(regVehFollData, longAdjustmentData);
  state LaneChanging
    entry:
    state = 3;
    during:
    data = min(regVehFollData, laneChangingData);
  (default) -> RegVehFoll
  LaneChanging -> RegVehFoll : [laneChangeDone]
  RegVehFoll -> LaneChanging [order 2] : [laneChangeStarted && ~laneChangeDone]
  RegVehFoll -> AdjForLaneChange [order 1] : [startAdjustment && ~laneChangeStarted]
  AdjForLaneChange -> LaneChanging : [laneChangeStarted==1]
  data: regVehFollData input; longAdjustmentData input; laneChangingData input; startAdjustment input size=1; data output; laneChangeStarted input; state output; laneChangeDone input

== stateflow chart full_maneuver_platoon_new_strategy/Fo/ControlChoice ==
  state RegVehFoll
    entry:
    state = 1;
    during:
    data = regVehFollData;
  state AdjForLaneChange
    entry:
    state = 2;
    during:
    data = min(regVehFollData, longAdjustmentData);
  state LaneChanging
    entry:
    state = 3;
    during:
    data = min(regVehFollData, laneChangingData);
  (default) -> RegVehFoll
  LaneChanging -> RegVehFoll : [laneChangeDone]
  RegVehFoll -> LaneChanging [order 2] : [laneChangeStarted && ~laneChangeDone]
  RegVehFoll -> AdjForLaneChange [order 1] : [startAdjustment && ~laneChangeStarted]
  AdjForLaneChange -> LaneChanging : [laneChangeStarted==1]
  data: regVehFollData input; longAdjustmentData input; laneChangingData input; startAdjustment input size=1; data output; laneChangeStarted input; state output; laneChangeDone input

== matlab function full_maneuver_platoon_new_strategy/Fo/MATLAB Function ==
  data: leader output Bus: vehStatesBus; ego input Bus: vehStatesBus; allVehicles input; indices output
function [leader, indices] = findLeader(ego, allVehicles)

nv = length(allVehicles);

leaderIdx = -1;

farAwayVehicle.X = ego.X + 10^4;
farAwayVehicle.Y = ego.Y;
farAwayVehicle.Xdot = ego.Xdot;
farAwayVehicle.u = 0;

leader = farAwayVehicle;

for n = 1:nv
    if allVehicles(n).X>ego.X && allVehicles(n).X<leader.X
        if abs(allVehicles(n).Y - ego.Y)<=2.7 % 1.8 (half lane) + 0.9 (half veh width)
            leader = allVehicles(n);
            leaderIdx=n;
        end
    end
end

indices = leaderIdx;

== stateflow chart full_maneuver_platoon_new_strategy/Fd/Vehicle Following During LC/Chart ==
  state VehFollowing
    during:
    u = uVehFoll;
    state = 0;
  state SpeedControl
    during:
    u = uVelControl;
    state = 1;
  (default) -> VehFollowing
  SpeedControl -> VehFollowing : [leaderWithinRange==1]
  VehFollowing -> SpeedControl : [leaderWithinRange==0]
  data: state output size=1; u output size=1; leaderWithinRange input size=1; uVehFoll input size=1; uVelControl input double

== matlab function full_maneuver_platoon_new_strategy/Lo/MATLAB Function ==
  data: leader output Bus: vehStatesBus; ego input Bus: vehStatesBus; allVehicles input; indices output
function [leader, indices] = findLeader(ego, allVehicles)

nv = length(allVehicles);

leaderIdx = -1;

farAwayVehicle.X = ego.X + 10^4;
farAwayVehicle.Y = ego.Y;
farAwayVehicle.Xdot = ego.Xdot;
farAwayVehicle.u = 0;

leader = farAwayVehicle;

for n = 1:nv
    if allVehicles(n).X>ego.X && allVehicles(n).X<leader.X
        if abs(allVehicles(n).Y - ego.Y)<=2.7 % 1.8 (half lane) + 0.9 (half veh width)
            leader = allVehicles(n);
            leaderIdx=n;
        end
    end
end

indices = leaderIdx;

== stateflow chart full_maneuver_platoon_new_strategy/Fo/Regular Vehicle Following/Chart ==
  state VehFollowing
    during:
    u = uVehFoll;
    state = 0;
  state SpeedControl
    during:
    u = uVelControl;
    state = 1;
  (default) -> VehFollowing
  SpeedControl -> VehFollowing : [leaderWithinRange==1]
  VehFollowing -> SpeedControl : [leaderWithinRange==0]
  data: state output size=1; u output size=1; leaderWithinRange input size=1; uVehFoll input size=1; uVelControl input double

== stateflow chart full_maneuver_platoon_new_strategy/Lo/Regular Vehicle Following/Chart ==
  state VehFollowing
    during:
    u = uVehFoll;
    state = 0;
  state SpeedControl
    during:
    u = uVelControl;
    state = 1;
  (default) -> VehFollowing
  SpeedControl -> VehFollowing : [leaderWithinRange==1]
  VehFollowing -> SpeedControl : [leaderWithinRange==0]
  data: state output size=1; u output size=1; leaderWithinRange input size=1; uVehFoll input size=1; uVelControl input double

== matlab function full_maneuver_platoon_new_strategy/p1/MATLAB Function ==
  data: leader output Bus: vehStatesBus; ego input Bus: vehStatesBus; allVehicles input; indices output; lcFlag input
function [leader, indices] = findLeader(ego, allVehicles, lcFlag)

nv = length(allVehicles);

leaderIdx = -1;

farAwayVehicle.X = ego.X + 10^4;
farAwayVehicle.Y = ego.Y;
farAwayVehicle.Xdot = ego.Xdot;
farAwayVehicle.u = 0;

leader = farAwayVehicle;

% For non lane changing vehicles, the leader is whoever is longitudinally
% closer and with any part of the body in the same lane
if ~lcFlag
    for n = 1:nv
        if allVehicles(n).X>ego.X && allVehicles(n).X<leader.X
            if abs(allVehicles(n).Y - ego.Y)<=2.7 % 1.8 (half lane) + 0.9 (half veh width)
                leader = allVehicles(n);
                leaderIdx=n;
            end
        end
    end
% For lane changing vehicles, we want to keep the original leader until the
% ego vehicle is out of the lane
else
    for n = 1:nv
        if allVehicles(n).X>ego.X && allVehicles(n).X<leader.X
            if abs(allVehicles(n).Y - ego.Y)<=1.9 % 1.8 (half lane) + 0.9 (half veh width)
                leader = allVehicles(n);
                leaderIdx=n;
            end
        end
    end
end

indices = leaderIdx;

== stateflow chart full_maneuver_platoon_new_strategy/Fd/Virtual Vehicle Following/Chart ==
  state VehFollowing
    during:
    u = uVehFoll;
    state = 0;
  state SpeedControl
    during:
    u = uVelControl;
    state = 1;
  (default) -> VehFollowing
  SpeedControl -> VehFollowing : [uVehFoll>=uVelControl]
  VehFollowing -> SpeedControl : [(velDiff>=0) && (uVehFoll<0)]
  data: state output size=1; u output size=1; velDiff input size=1; uVelControl input double; uVehFoll input size=1

== stateflow chart full_maneuver_platoon_new_strategy/p1/Regular Vehicle Following/Chart ==
  state VehFollowing
    during:
    u = uVehFoll;
    state = 0;
  state SpeedControl
    during:
    u = uVelControl;
    state = 1;
  (default) -> VehFollowing
  SpeedControl -> VehFollowing : [leaderWithinRange==1]
  VehFollowing -> SpeedControl : [leaderWithinRange==0]
  data: state output size=1; u output size=1; leaderWithinRange input size=1; uVehFoll input size=1; uVelControl input double

== stateflow chart full_maneuver_platoon_new_strategy/p1/Vehicle Following During LC/Chart ==
  state VehFollowing
    during:
    u = uVehFoll;
    state = 0;
  state SpeedControl
    during:
    u = uVelControl;
    state = 1;
  (default) -> VehFollowing
  SpeedControl -> VehFollowing : [leaderWithinRange==1]
  VehFollowing -> SpeedControl : [leaderWithinRange==0]
  data: state output size=1; u output size=1; leaderWithinRange input size=1; uVehFoll input size=1; uVelControl input double

== stateflow chart full_maneuver_platoon_new_strategy/Lo/Vehicle Following During LC/Chart ==
  state VehFollowing
    during:
    u = uVehFoll;
    state = 0;
  state SpeedControl
    during:
    u = uVelControl;
    state = 1;
  (default) -> VehFollowing
  SpeedControl -> VehFollowing : [leaderWithinRange==1]
  VehFollowing -> SpeedControl : [leaderWithinRange==0]
  data: state output size=1; u output size=1; leaderWithinRange input size=1; uVehFoll input size=1; uVelControl input double

== stateflow chart full_maneuver_platoon_new_strategy/Ld/Vehicle Following During LC/Chart ==
  state VehFollowing
    during:
    u = uVehFoll;
    state = 0;
  state SpeedControl
    during:
    u = uVelControl;
    state = 1;
  (default) -> VehFollowing
  SpeedControl -> VehFollowing : [leaderWithinRange==1]
  VehFollowing -> SpeedControl : [leaderWithinRange==0]
  data: state output size=1; u output size=1; leaderWithinRange input size=1; uVehFoll input size=1; uVelControl input double

== stateflow chart full_maneuver_platoon_new_strategy/Ld/Virtual Vehicle Following/Chart ==
  state VehFollowing
    during:
    u = uVehFoll;
    state = 0;
  state SpeedControl
    during:
    u = uVelControl;
    state = 1;
  (default) -> VehFollowing
  SpeedControl -> VehFollowing : [uVehFoll>=uVelControl]
  VehFollowing -> SpeedControl : [(velDiff>=0) && (uVehFoll<0)]
  data: state output size=1; u output size=1; velDiff input size=1; uVelControl input double; uVehFoll input size=1

== stateflow chart full_maneuver_platoon_new_strategy/Lo/Virtual Vehicle Following/Chart ==
  state VehFollowing
    during:
    u = uVehFoll;
    state = 0;
  state SpeedControl
    during:
    u = uVelControl;
    state = 1;
  (default) -> VehFollowing
  SpeedControl -> VehFollowing : [uVehFoll>=uVelControl]
  VehFollowing -> SpeedControl : [(velDiff>=0) && (uVehFoll<0)]
  data: state output size=1; u output size=1; velDiff input size=1; uVelControl input double; uVehFoll input size=1

== stateflow chart full_maneuver_platoon_new_strategy/Fo/Vehicle Following During LC/Chart ==
  state VehFollowing
    during:
    u = uVehFoll;
    state = 0;
  state SpeedControl
    during:
    u = uVelControl;
    state = 1;
  (default) -> VehFollowing
  SpeedControl -> VehFollowing : [leaderWithinRange==1]
  VehFollowing -> SpeedControl : [leaderWithinRange==0]
  data: state output size=1; u output size=1; leaderWithinRange input size=1; uVehFoll input size=1; uVelControl input double

== stateflow chart full_maneuver_platoon_new_strategy/Fo/Virtual Vehicle Following/Chart ==
  state VehFollowing
    during:
    u = uVehFoll;
    state = 0;
  state SpeedControl
    during:
    u = uVelControl;
    state = 1;
  (default) -> VehFollowing
  SpeedControl -> VehFollowing : [uVehFoll>=uVelControl]
  VehFollowing -> SpeedControl : [(velDiff>=0) && (uVehFoll<0)]
  data: state output size=1; u output size=1; velDiff input size=1; uVelControl input double; uVehFoll input size=1

== stateflow chart full_maneuver_platoon_new_strategy/p2/ControlChoice ==
  state RegVehFoll
    entry:
    state = 1;
    during:
    data = regVehFollData;
  state AdjForLaneChange
    entry:
    state = 2;
    during:
    if leaderInRange
    data = min(regVehFollData, longAdjustmentData);
    else
    data = longAdjustmentData;
    end
  state LaneChanging
    entry:
    state = 3;
    during:
    if leaderInRange
    data = min(regVehFollData, laneChangingData);
    else
    data = laneChangingData;
    end
  (default) -> RegVehFoll
  LaneChanging -> RegVehFoll : [laneChangeDone]
  RegVehFoll -> LaneChanging [order 2] : [laneChangeStarted && ~laneChangeDone]
  RegVehFoll -> AdjForLaneChange [order 1] : [startAdjustment && ~laneChangeStarted]
  AdjForLaneChange -> LaneChanging : [laneChangeStarted]
  data: regVehFollData input; longAdjustmentData input; laneChangingData input; startAdjustment input size=1; data output; laneChangeStarted input; state output; laneChangeDone input; leaderInRange input

== matlab function full_maneuver_platoon_new_strategy/p2/MATLAB Function ==
  data: leader output Bus: vehStatesBus; ego input Bus: vehStatesBus; allVehicles input; indices output; lcFlag input
function [leader, indices] = findLeader(ego, allVehicles, lcFlag)

nv = length(allVehicles);

leaderIdx = -1;

farAwayVehicle.X = ego.X + 10^4;
farAwayVehicle.Y = ego.Y;
farAwayVehicle.Xdot = ego.Xdot;
farAwayVehicle.u = 0;

leader = farAwayVehicle;

% For non lane changing vehicles, the leader is whoever is longitudinally
% closer and with any part of the body in the same lane
if ~lcFlag
    for n = 1:nv
        if allVehicles(n).X>ego.X && allVehicles(n).X<leader.X
            if abs(allVehicles(n).Y - ego.Y)<=2.7 % 1.8 (half lane) + 0.9 (half veh width)
                leader = allVehicles(n);
                leaderIdx=n;
            end
        end
    end
% For lane changing vehicles, we want to keep the original leader until the
% ego vehicle is out of the lane
else
    for n = 1:nv
        if allVehicles(n).X>ego.X && allVehicles(n).X<leader.X
            if abs(allVehicles(n).Y - ego.Y)<=1.9 % 1.8 (half lane) + 0.9 (half veh width)
                leader = allVehicles(n);
                leaderIdx=n;
            end
        end
    end
end

indices = leaderIdx;
